simulink model "Model"  (R2024b)
settings: Solver=VariableStepAuto  StartTime=0.0  StopTime=2000  RelTol=1e-3
values from neighbouring files (symbols this model uses):
  A = sys_3dof_w2v.A    [Sys.m]
  Alqg = sys_zv.A - sys_zv.B*K - L*sys_zv.C    [Decoupled_LQG.m]    (also in SISO_LQG.m = Gv.A - Gv.B*K - L*Gv.C)
  B = sys_3dof_w2v.B    [Sys.m]
  Blqg = L    [Decoupled_LQG.m]    (also in SISO_LQG.m)
  C = sys_3dof_w2v.C    [Sys.m]
  Clqg = -K    [Decoupled_LQG.m]    (also in SISO_LQG.m)
  D = sys_3dof_w2v.D    [Sys.m]
  Dlqg = zeros(3, 3)    [Decoupled_LQG.m]    (also in SISO_LQG.m = zeros(1, 1))
  Ts = 1/fs    (= 0.0001)    [Sys.m]
  Tu = [ 1  1  0 ... (first row only)    [Decoupled_LQG.m]    (also in SISO_LQG.m)
  Ty = [   0.5  0    0.5  0 ... (first row only)    [Decoupled_LQG.m]    (also in SISO_LQG.m)
undefined symbols (not defined in the file or in its folder): Ag, Ahims, Ans, Bg, Bhims, Bns, C1, C2, C3, Cg, Chims, Cns, Dg, Dhims, Dns
libraries: simulink x4, slpidlib x1
settings Model: Creator=yangshuyun  LastModifiedBy=yangshuyun

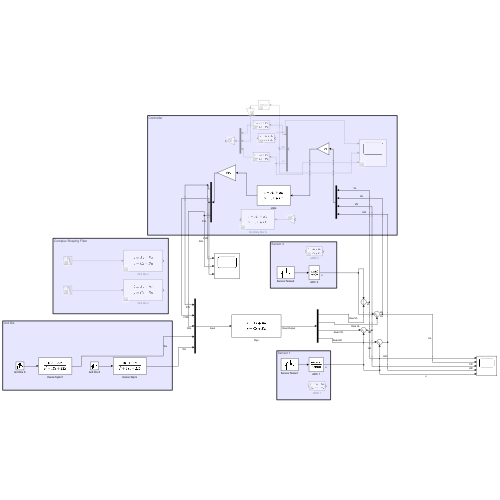
[thumbnail: Simulink's stored preview of the top-level diagram]
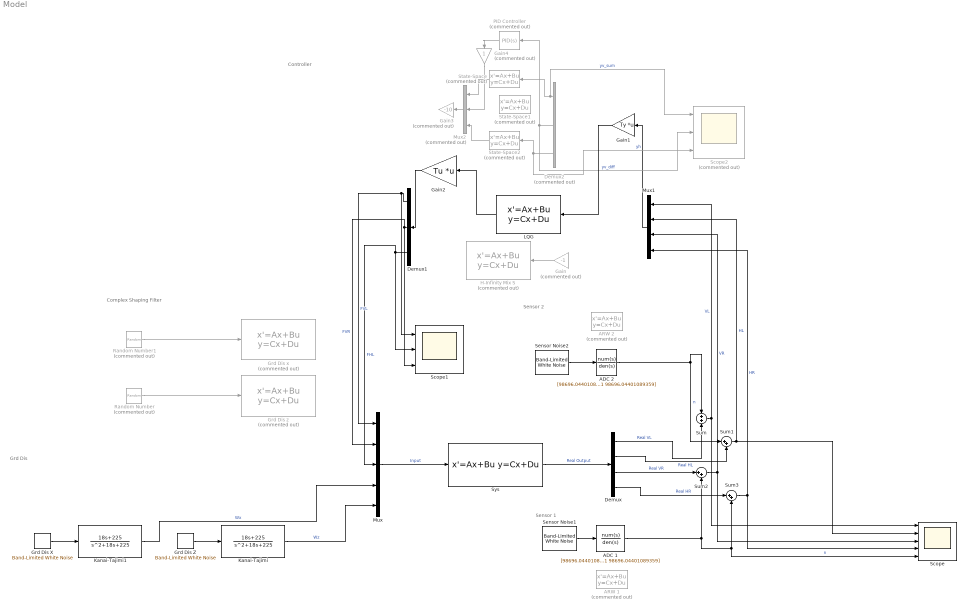
== system Model ==
  note: Controller
  note: Sensor 2
  note: Sensor 1
  note: Grd Dis
  note: Complex Shaping Filter
  ADC 1 : TransferFcn  Numerator=[98696.04401089359]  Denominator=[1 439.822971502571 98696.04401089359]
  ADC 2 : TransferFcn  Numerator=[98696.04401089359]  Denominator=[1 439.822971502571 98696.04401089359]
  ARW 1 : StateSpace  Commented=on  A=Ans  B=Bns  C=Cns  D=Dns  InitialCondition=0
  ARW 2 : StateSpace  Commented=on  A=Ans  B=Bns  C=Cns  D=Dns  InitialCondition=0
  Demux : Demux
  Demux1 : Demux  Outputs=3
  Demux2 : Demux  Commented=on  Outputs=3
  Gain : Gain  Commented=on  Gain=-1
  Gain1 : Gain  Gain=Ty  Multiplication=Matrix(K*u)
  Gain2 : Gain  Gain=Tu  Multiplication=Matrix(K*u)
  Gain3 : Gain  Commented=on  Gain=-10
  Gain4 : Gain  Commented=on
  Grd Dis X : simulink/Sources/Band-Limited White Noise  Cov=[1e-14]  Ts=Ts  seed=[619]
  Grd Dis Z : simulink/Sources/Band-Limited White Noise  Cov=[1e-14]  Ts=Ts  seed=[42]
  Grd Dis x : StateSpace  Commented=on  A=Ag  B=Bg  C=Cg  D=Dg  InitialCondition=0
  Grd Dis z : StateSpace  Commented=on  A=Ag  B=Bg  C=Cg  D=Dg  InitialCondition=0
  H-Infinity Mix S : StateSpace  Commented=on  A=Ahims  B=Bhims  C=Chims  D=Dhims  InitialCondition=0
  Kanai-Tajimi : TransferFcn  Numerator=[18, 225]  Denominator=[1, 18, 225]
  Kanai-Tajimi1 : TransferFcn  Numerator=[18, 225]  Denominator=[1, 18, 225]
  LQG : StateSpace  A=Alqg  B=Blqg  C=Clqg  D=Dlqg  InitialCondition=0
  Mux : Mux  Inputs=5
  Mux1 : Mux
  Mux2 : Mux  Commented=on  Inputs=3
  PID Controller : slpidlib/PID Controller  Commented=on  Controller=PID  Form=Parallel  TimeDomain=Continuous-time  UseExternalTs=off  SampleTime=-1  IntegratorMethod=Forward Euler  FilterMethod=Forward Euler  ControllerParametersSource=internal  P=0  I=456.839263048745  UseKiTs=off  D=0  UseExternalDerivativeSource=off  N=100  UseFilter=on  TunerSelectOption=Transfer Function Based (PID Tuner App)  InitialConditionSource=internal  InitialConditionForIntegrator=0  InitialConditionForFilter=0  DifferentiatorICPrevScaledInput=0  ExternalReset=none  TrackingMode=off  Kt=1  LimitOutput=off  SatLimitsSource=internal  UpperSaturationLimit=inf  LowerSaturationLimit=-inf  LinearizeAsGain=on  AntiWindupMode=none  Kb=1  LimitIntegrator=off  UpperIntegratorSaturationLimit=inf  LowerIntegratorSaturationLimit=-inf  POutMin=[]  POutMax=[]  IOutMin=[]  IOutMax=[]  DOutMin=[]  DOutMax=[]  NOutMin=[]  NOutMax=[]  SumOutMin=[]  SumOutMax=[]  SaturationOutMin=[]  SaturationOutMax=[]  PParamMin=[]  PParamMax=[]  IParamMin=[]  IParamMax=[]  DParamMin=[]  DParamMax=[]  NParamMin=[]  NParamMax=[]  KbParamMin=[]  KbParamMax=[]  KtParamMin=[]  KtParamMax=[]  KbOutMin=[]  KbOutMax=[]  KtOutMin=[]  KtOutMax=[]  IntegratorOutMin=[]  IntegratorOutMax=[]  FilterOutMin=[]  FilterOutMax=[]  SumI1OutMin=[]  SumI1OutMax=[]  SumI2OutMin=[]  SumI2OutMax=[]  SumI3OutMin=[]  SumI3OutMax=[]  SumI4OutMin=[]  SumI4OutMax=[]  SumDOutMin=[]  SumDOutMax=[]  DifferentiatorOutMin=[]  DifferentiatorOutMax=[]  FilterDiffOutCoefMin=[]  FilterDiffOutCoefMax=[]  ReciprocalOutMin=[]  ReciprocalOutMax=[]  SumDenOutMin=[]  SumDenOutMax=[]  SumNumOutMin=[]  SumNumOutMax=[]  DivideOutMin=[]  DivideOutMax=[]  UdiffTsProdOutMin=[]  UdiffTsProdOutMax=[]  NTsProdOutMin=[]  NTsProdOutMax=[]  UintegralTsProdOutMin=[]  UintegralTsProdOutMax=[]  UngainTsProdOutMin=[]  UngainTsProdOutMax=[]  ClampingZeroOutDataTypeStr=Inherit: Inherit via back propagation  ClampingZeroOutMin=[]  ClampingZeroOutMax=[]  FilterDenConstantOutDataTypeStr=Inherit: Inherit via back propagation  FilterDenConstantOutMin=[]  FilterDenConstantOutMax=[]  PCopyOutDataTypeStr=Inherit: Inherit via back propagation  PCopyOutMin=[]  PCopyOutMax=[]  NCopyOutDataTypeStr=Inherit: Inherit via back propagation  NCopyOutMin=[]  NCopyOutMax=[]  IntegratorContinuousStateAttributes=''  IntegratorStateMustResolveToSignalObject=off  IntegratorRTWStateStorageClass=Auto  FilterContinuousStateAttributes=''  FilterStateMustResolveToSignalObject=off  FilterRTWStateStorageClass=Auto  ParallelPVariant=InternalParameters  IdealPVariant=Disabled  IVariant=InternalParameters  DVariant=InternalParameters  IntegratorVariant=Continuous  SatVariant=Disabled  AWVariant=Passthrough  PCopyVariant=Disabled  TRVariant=Disabled  FdbkBlocksVariant=Forward  IdealPFdbkVariant=Disabled  SatFdbkVariant=Disabled  DerivativeFilterVariant=ContFilter  NVariant=InternalParameters  NCopyVariant=Disabled  FilterICVariant=InternalICsFilter  IntegratorICVariant=InternalICs  ExternalResetVariant=Disabled  TRSumVariant=Passthrough  SumFdbkVariant=Disabled  SumVariant=Sum_PID  TsampFilterVariant=InternalTs  TsampNgainVariant=Passthrough  TsampIntegralVariant=Disabled_SignalSpec  ExternalSaturationOutDataTypeStr=Inherit: Same as second input  DerivativeSourceVariant=ErrorSignal  PreIntVariant=InternalPreInt
  Random Number : RandomNumber  Commented=on  Variance=100/Ts  Seed=42  SampleTime=Ts
  Random Number1 : RandomNumber  Commented=on  Variance=100/Ts  SampleTime=Ts
  Scope : Scope  NumInputPorts=5
  Scope1 : Scope  NumInputPorts=3
  Scope2 : Scope  Commented=on  NumInputPorts=3
  Sensor Noise1 : simulink/Sources/Band-Limited White Noise  Cov=1e-15  Ts=Ts  seed=[23341]
  Sensor Noise2 : simulink/Sources/Band-Limited White Noise  Cov=1e-15  Ts=Ts  seed=[114]
  State-Space : StateSpace  Commented=on  A=C1.A  B=C1.B  C=C1.C  D=C1.D  InitialCondition=0
  State-Space1 : StateSpace  Commented=on  A=C2.A  B=C2.B  C=C2.C  D=C2.D  InitialCondition=0
  State-Space2 : StateSpace  Commented=on  A=C3.A  B=C3.B  C=C3.C  D=C3.D  InitialCondition=0
  Sum : Sum  Inputs=+|+
  Sum1 : Sum  Inputs=|++
  Sum2 : Sum  Inputs=|++
  Sum3 : Sum  Inputs=|++
  Sys : StateSpace  A=A  B=B  C=C  D=D  InitialCondition=0
  wires:
  Mux/1 -> Sys/1  "Input"
  Sys/1 -> Demux/1  "Real Output"
  Demux/4 -> Sum3/1  "Real HR"
  Demux/3 -> Sum2/1  "Real VR"
  Demux/2 -> Sum1/2  "Real HL"
  Demux/1 -> Sum/2  "Real VL"
  Demux1/1 -> Mux/1, Scope1/1  "FVL"
  Demux1/2 -> Mux/2, Scope1/3  "FVR"
  Demux1/3 -> Mux/3, Scope1/2  "FHL"
  Random Number1/1 -> Grd Dis x/1
  Random Number/1 -> Grd Dis z/1
  Sum/1 -> Mux1/1, Scope/1  "VL"
  Sum1/1 -> Scope/2, Mux1/2  "HL"
  Sum2/1 -> Scope/3, Mux1/3  "VR"
  Sum3/1 -> Scope/4, Mux1/4  "HR"
  Grd Dis Z/1 -> Kanai-Tajimi/1
  Kanai-Tajimi1/1 -> Mux/4  "Wx"
  Grd Dis X/1 -> Kanai-Tajimi1/1
  Kanai-Tajimi/1 -> Mux/5  "Wz"
  Sensor Noise1/1 -> ADC 1/1
  Sensor Noise2/1 -> ADC 2/1
  ADC 2/1 -> Sum/1, Sum1/1  "n"
  ADC 1/1 -> Scope/5, Sum3/2, Sum2/2  "n"
  Gain/1 -> H-Infinity Mix S/1
  Mux1/1 -> Gain1/1
  State-Space/1 -> Mux2/1
  Demux2/1 -> Scope2/1, State-Space/1  "yv_sum"
  Demux2/3 -> State-Space2/1, Scope2/3  "yh"
  Gain2/1 -> Demux1/1
  Demux2/2 -> PID Controller/1, Scope2/2  "yv_diff"
  Mux2/1 -> Gain3/1
  State-Space2/1 -> Mux2/3
  PID Controller/1 -> Gain4/1
  Gain4/1 -> Mux2/2
  LQG/1 -> Gain2/1
  Gain1/1 -> LQG/1
